simulink model "lab5"  (R2020b)
settings: Solver=ode45  StartTime=0.0  StopTime=135  RelTol=1e-3  EnableMultiTasking=on
values from neighbouring files (symbols this model uses):
  alpha1 = 7.84e-3    (= 0.00784)    [lab5m.m]    (also in obg_reg.m = hyperspherical(theta1))
  alpha2 = 9.09e-3    (= 0.00909)    [lab5m.m]    (also in obg_reg.m = alpha1.*[1;exp(j*theta2)])
  beta = 2334    [initHW4.m]    (also in initLab4.m; lab5m.m = 0.225)
  C = [1, 0]    [initHW4.m]    (also in initLab4.m = [1, 0, 0, 0; lab5m.m = [0 1])
  g = 9.81    [initLab4.m]    (also in lab5m.m = 981)
  gammaa = 1    [initHW4.m]    (also in lab5m.m)
  K1 = Kd(:,1:n)    [tsd.m]
  K2 = Kd(:,n+1:n+q)    [tsd.m]
  noise = 0    [lab5m.m]
  phia = 1    [initHW4.m]    (also in lab5m.m)
  T = min(Ts / 20 * (nOrder + 1),      pi / (5 * TbetaMax))    [initHW4.m]    (also in initLab4.m = 0.01; lab5m.m = 0.1)
  ue = alpha1*sqrt(2*g*xe1)/beta    [lab5m.m]
  xa0 = -(ue+K1*xe)/K2    [lab5m.m]
  xe = [xe1;xe2]    [lab5m.m]
libraries: simulink x2
settings Model: Creator=RJV  LastModifiedBy=rjv
settings DataIOCC: LimitDataPoints=on  SaveFormat=Array  SignalLoggingSaveFormat=ModelDataLogs  ReturnWorkspaceOutputs=off
settings OptimizationCC: ExpressionDepthLimit=2147483647  LifeSpan=inf
settings DebuggingCC: UnderspecifiedInitializationDetection=Classic  MergeDetectMultiDrivingBlocksExec=none  SolverPrmCheckMsg=warning  FcnCallInpInsideContextMsg=warning  StateNameClashWarn=warning  SFUnexpectedBacktrackingDiag=warning  SFNoUnconditionalDefaultTransitionDiag=warning  SFExecutionAtInitializationDiag=none  ArithmeticOperatorsInVariantConditions=warning
settings HardwareCC: ProdBitPerPointer=32  ProdBitPerSizeT=32  ProdBitPerPtrDiffT=32  ProdLargestAtomicFloat=None  ProdIntDivRoundTo=Undefined  ProdEndianess=Unspecified  ProdWordSize=32  ProdHWDeviceType=32-bit Generic
settings ModelReferenceCC: PropagateSignalLabelsOutOfModel=off
settings SFSimCC: SimUseLocalCustomCode=off  CustomCodeUndefinedFunction=UseInterfaceOnly
settings RTWCC: RTWUseLocalCustomCode=off
settings CodeAppCC: StateflowObjectComments=on
settings GRTTargetCC: TargetLangStandard=C89/C90 (ANSI)  CombineOutputUpdateFcns=off  GRTInterface=on
settings ConfigComp: CovMetricSettings=dw  CovSaveCumulativeToWorkspaceVar=on  CovSaveSingleToWorkspaceVar=on  CovExternalEMLEnable=off  CovSFcnEnable=off

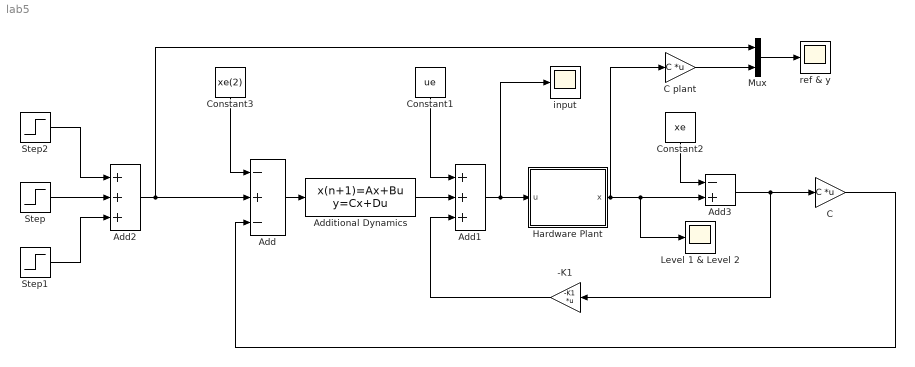
== system lab5 ==
  -K1 : Gain  Gain=-K1  Multiplication=Matrix(K*u)  SampleTime=T
  Add : Sum  Inputs=-+-  SampleTime=T
  Add1 : Sum  Inputs=+++  SampleTime=T
  Add2 : Sum  Inputs=+++  SampleTime=T
  Add3 : Sum  Inputs=-+  SampleTime=T
  Additional Dynamics : DiscreteStateSpace  A=phia  B=gammaa  C=K2  D=0  InitialCondition=xa0  SampleTime=T
  C : Gain  Gain=C  Multiplication=Matrix(K*u)  SampleTime=T
  C plant : Gain  Gain=C  Multiplication=Matrix(K*u)  SampleTime=T
  Constant1 : Constant  Value=ue
  Constant2 : Constant  Value=xe
  Constant3 : Constant  Value=xe(2)
  Hardware Plant : Subsystem
  Level 1 & Level 2 : Scope
  Mux : Mux  Inputs=2
  Step : Step  Time=45  After=3  SampleTime=0
  Step1 : Step  Time=90  After=-3  SampleTime=0
  Step2 : Step  Time=0  After=12  SampleTime=0
  input : Scope
  ref & y : Scope
  wires:
  Add/1 -> Additional Dynamics/1
  Additional Dynamics/1 -> Add1/2
  Constant3/1 -> Add/1
  Step2/1 -> Add2/1
  Step/1 -> Add2/2
  Step1/1 -> Add2/3
  Add2/1 -> Add/2, Mux/1
  Constant1/1 -> Add1/1
  Add1/1 -> input/1, Hardware Plant/1(u)
  -K1/1 -> Add1/3
  Hardware Plant/1(x) -> C plant/1, Add3/2, Level 1 & Level 2/1
  Constant2/1 -> Add3/1
  Add3/1 -> C/1, -K1/1
  C/1 -> Add/3
  C plant/1 -> Mux/2
  Mux/1 -> ref & y/1

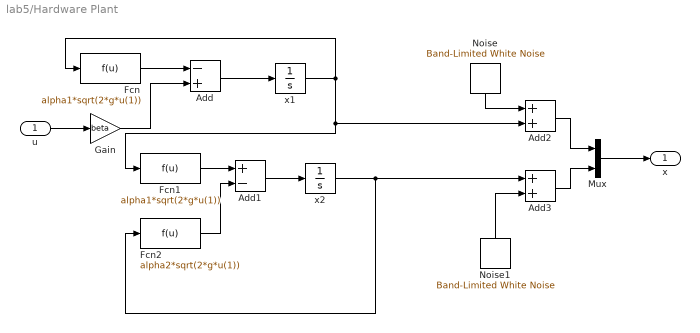
== system lab5/Hardware Plant ==
  u : Inport
  Add : Sum  Inputs=-+
  Add1 : Sum  Inputs=+-
  Add2 : Sum
  Add3 : Sum
  Fcn : Fcn  Expr=alpha1*sqrt(2*g*u(1))
  Fcn1 : Fcn  Expr=alpha1*sqrt(2*g*u(1))
  Fcn2 : Fcn  Expr=alpha2*sqrt(2*g*u(1))
  Gain : Gain  Gain=beta
  Mux : Mux  Inputs=2
  Noise : simulink/Sources/Band-Limited White Noise  Cov=noise*0.001  Ts=T  seed=[23341]
  Noise1 : simulink/Sources/Band-Limited White Noise  Cov=noise*0.001  Ts=T  seed=[14332]
  x1 : Integrator
  x2 : Integrator
  x : Outport
  wires:
  Add/1 -> x1/1
  Fcn/1 -> Add/1
  x1/1 -> Fcn/1, Fcn1/1, Add2/2
  Gain/1 -> Add/2
  Add1/1 -> x2/1
  Fcn1/1 -> Add1/1
  x2/1 -> Fcn2/1, Add3/1
  Fcn2/1 -> Add1/2
  Mux/1 -> x/1
  Noise1/1 -> Add3/2
  Noise/1 -> Add2/1
  Add2/1 -> Mux/1
  Add3/1 -> Mux/2
  u/1 -> Gain/1
